simulink model "run_quadrotor_2020a"  (R2020a)
settings: Solver=ode23  StartTime=0.0  StopTime=60  FixedStep=10/1000  MaxStep=0.01  MinStep=1/1000  RelTol=1e-5  EnableMultiTasking=on
InitFcn:
  | addpath('display/')
  | addpath('parameters/')
  | addpath('quadrotor_model')
  | addpath('tools/')
  | addpath('libs/RealTima_Pacer')
  | aerosonde_parameters
  | simulation_parameters
model workspace (MAT data in the model file):
  D1_podbor1 = 902.0676
  D1_podbor_psi = 334.133298018
  D1_podbor_y = 97.9069
  D_podbor_x = 10
  D_podbor_z = 10
  I1_podbor1 = 320.9285
  I1_podbor_psi = 2.71828630961
  I1_podbor_y = 0.6752
  I_podbor_x = 50
  I_podbor_z = 50
  P1_podbor1 = 7509.4
  P1_podbor_psi = 848.547345881
  P1_podbor_y = 264.9363
  P_podbor_x = 50
  P_podbor_z = 50
  theta_1_P_param = Simulink.Parameter
  theta_1_P_param.Value = 1
  theta_1_P_param.DataType = 'auto'
  theta_1_P_param.Dimensions = [1 1]
  theta_1_P_paramCopy = Simulink.Parameter
  theta_1_P_paramCopy.Value = 1
  theta_1_P_paramCopy.DataType = 'auto'
  theta_1_P_paramCopy.Dimensions = [1 1]
undefined symbols (not defined in the file or in its folder): drawQuadrotor, filter_freq, ln, MAV, plotmavstatevariables, setup_pid
libraries: simulink x11, checkpacklib x5, dspsigattribs x2, realtime_pacer_lib x1
(part 1 of 2)
settings Model: PacingRate=0.160000  ParameterArgumentNames=theta_1_P_param  OrderedModelArguments=off  Creator=beard  LastModifiedBy=Tamer
settings SolverCC: ZeroCrossControl=DisableAll
settings DataIOCC: LimitDataPoints=on  SaveFormat=Array  ReturnWorkspaceOutputsName=SDOSimTest_Log
settings OptimizationCC: ExpressionDepthLimit=2147483647  InitFltsAndDblsToZero=on  LifeSpan=inf  SimCompilerOptimization=on
settings DebuggingCC: ReadBeforeWriteMsg=DisableAll  WriteAfterWriteMsg=DisableAll  WriteAfterReadMsg=DisableAll  MergeDetectMultiDrivingBlocksExec=none  SolverPrmCheckMsg=warning  MultiTaskDSMMsg=none  IntegerOverflowMsg=none  FcnCallInpInsideContextMsg=warning  AllowSymbolicDim=off  StateNameClashWarn=warning  SFUnexpectedBacktrackingDiag=warning  SFNoUnconditionalDefaultTransitionDiag=warning  SFExecutionAtInitializationDiag=none  IntegerSaturationMsg=none  ArithmeticOperatorsInVariantConditions=warning
settings ModelReferenceCC: UpdateModelReferenceTargets=IfOutOfDate  PropagateSignalLabelsOutOfModel=off
settings SFSimCC: SFSimEcho=off  SimCtrlC=off  SimUseLocalCustomCode=off  CustomCodeUndefinedFunction=UseInterfaceOnly
settings RTWCC: RTWUseLocalCustomCode=off
settings CodeAppCC: StateflowObjectComments=on
settings GRTTargetCC: TargetLangStandard=C89/C90 (ANSI)  CombineOutputUpdateFcns=off  GRTInterface=on
settings ConfigComp: CovMetricSettings=dw  CovSaveCumulativeToWorkspaceVar=on  CovSaveSingleToWorkspaceVar=on  CovExternalEMLEnable=off  CovSFcnEnable=off

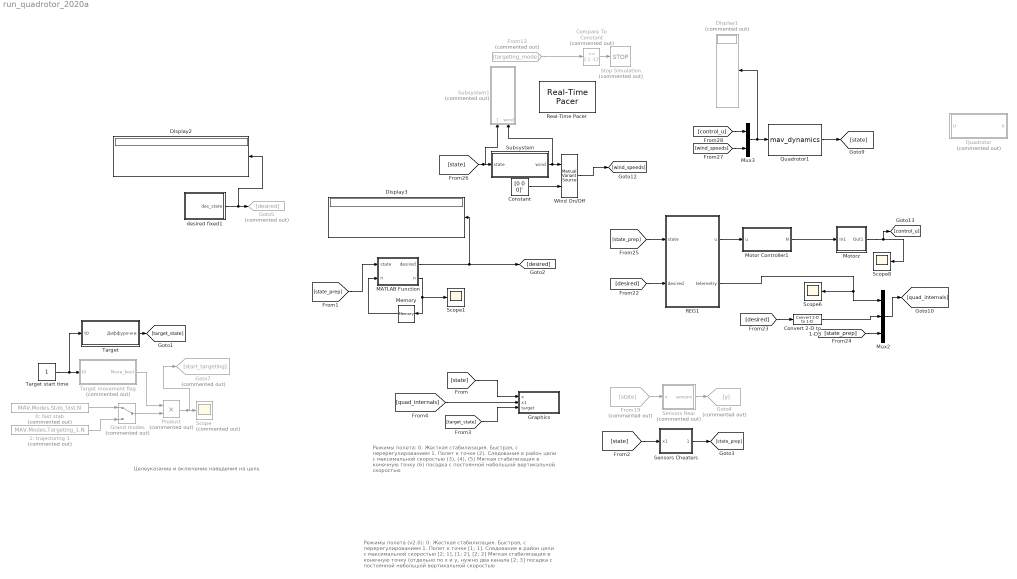
== system run_quadrotor_2020a ==
  note: Целеуказание и включение наведения на цель
  note: Режимы полета:
      | 0. Жесткая стабилизация. Быстрая, с перерегулированием
      | 1. Полет к точке
      |     (2). Следование в район цели с максимальной скоростью
      |     (3), (4), (5) Мягкая стабилизация в конечную точку
      |     (6) посадка с постоянной небольшой вертикальной   скоростью
  note: Режимы полета (v2.0):
      | 0. Жесткая стабилизация. Быстрая, с перерегулированием
      | 1. Полет к точке
      |     [1; 1]. Следование в район цели с максимальной скоростью
      |     [2; 1], [1; 2], [2; 2] Мягкая стабилизация в конечную точку (отдельно по х и у, нужно два канала
      |     [2; 3] посадка с постоянной небольшой вертикальной   скоростью
  0: fast stab : Constant  Commented=on  Value=MAV.Modes.Stab_fast.N
  1: trajectoring 1 : Constant  Commented=on  Value=MAV.Modes.Targeting_1.N
  Compare To Constant : simulink/Logic and Bit Operations/Compare To Constant  Commented=on  relop===  const=[-1 -1]'  OutDataTypeStr=boolean
  Constant : Constant  Value=[0 0 0]'
  Convert 2-D to 1-D3 : dspsigattribs/Convert 2-D to 1-D
      settings: SourceProductBaseCode=DS
  Display1 : Display  Commented=on
  Display2 : Display
  Display3 : Display
  From13 : From  Commented=on  GotoTag=targeting_mode
  From19 : From  Commented=on  GotoTag=state
  Goto4 : Goto  Commented=on  GotoTag=y
  Goto5 : Goto  Commented=on  GotoTag=desired
  Goto7 : Goto  Commented=on  GotoTag=start_targeting
  Grand modes : ManualSwitch  Commented=on
  Graphics : Subsystem
      mask Display: image(imread('../chap2/tv.jpg'))
  MATLAB Function : MATLAB Function  TreatAsAtomicUnit=on
  Memory : Memory
  Motor Controller1 : MATLAB Function  TreatAsAtomicUnit=on
  Motorz : Subsystem
  Mux2 : Mux  Inputs=3
  Mux3 : Mux  Inputs=2
  Product : Product  Commented=on
  Quadrotor : Subsystem  Commented=on
  Quadrotor1 : S-Function  FunctionName=mav_dynamics  Parameters=MAV  SFunctionDeploymentMode=off  EnableBusSupport=off
  REG1 : Subsystem
  Real-Time Pacer : realtime_pacer_lib/Real-Time Pacer  simTimePerRealTime=1
  Scope : Scope  Commented=on
  Scope1 : Scope
  Scope6 : Scope
  Scope8 : Scope
  Sensors Cheaters : Subsystem
  Sensors Real : Subsystem  Commented=on
  Stop Simulation : Stop  Commented=on
  Subsystem : Subsystem
  Subsystem1 : Subsystem  Commented=on
  Target : Subsystem
  Target movement flag : Subsystem  Commented=on
  Target start time : Constant
  Wind On/Off : simulink/Signal Routing/Manual Variant Source  NumChoices=2  LabelModeActiveChoice=V_1
  desired fixed1 : MATLAB Function  TreatAsAtomicUnit=on
  wires:
  Target/1("Диффурочки ") -> [target_state]
  0: fast stab/1 -> Grand modes/1
  1: trajectoring 1/1 -> Grand modes/2
  Grand modes/1 -> Product/2
  Target movement flag/1(Move_bool) -> Product/1
  Product/1 -> Goto7/1, Scope/1
  [state] -> Graphics/1(x)
  [target_state] -> Graphics/3(target)
  Sensors Cheaters/1(sensors) -> [state_prep]
  [quad_internals] -> Graphics/2(x1)
  Compare To Constant/1 -> Stop Simulation/1
  From13/1 -> Compare To Constant/1
  Target start time/1 -> Target/1(t0), Target movement flag/1(t0)
  Sensors Real/1(sensors) -> Goto4/1
  From19/1 -> Sensors Real/1("x ")
  [state] -> Sensors Cheaters/1(x1)
  [state_prep] -> Mux2/3
  [desired] -> Convert 2-D to 1-D3/1
  Mux2/1 -> [quad_internals]
  [desired] -> REG1/2(desired)
  REG1/2(telemetry) -> Mux2/1, Scope6/1
  [state_prep] -> REG1/1(state)
  Convert 2-D to 1-D3/1 -> Mux2/2
  REG1/1(u) -> Motor Controller1/1(u)
  Motor Controller1/1(N) -> Motorz/1(In1)
  Motorz/1(Out1) -> [control_u], Scope8/1
  [state] -> Subsystem1/1(state), Subsystem/1(state)
  Subsystem/1(wind) -> Subsystem1/2(wind), Wind On/Off/1
  [control_u] -> Mux3/1
  [wind_speeds] -> Mux3/2
  Mux3/1 -> Display1/1, Quadrotor1/1
  Quadrotor1/1 -> [state]
  desired fixed1/1(des_state) -> Display2/1, Goto5/1
  Constant/1 -> Wind On/Off/2
  Wind On/Off/1 -> [wind_speeds]
  [state_prep] -> MATLAB Function/1(state)
  MATLAB Function/1(desired) -> Display3/1, [desired]
  MATLAB Function/2(n) -> Scope1/1, Memory/1
  Memory/1 -> MATLAB Function/2("n ")

== system run_quadrotor_2020a/Graphics ==
  note: 2. Дежрать окно с дерьмом в фокусе нахуй мое уважение
  note: 1. Переключиться на другое окно, затем переключить фокус обратно
  note: Attention!!! Для динамического изменения положения камеры (слежение за квадром) необходимо:
  x : Inport
  x1 : Inport  Port=2
  target : Inport  Port=3
  Clock : Clock
  Mux : Mux
  drawQuadrotor : MATLABFcn  MATLABFcn=drawQuadrotor(u)  OutputDimensions=0  SampleTime=0
  plotStateVariables : MATLABFcn  MATLABFcn=plotmavstatevariables(u)  OutputDimensions=0
  wires:
  x/1 -> Mux/1
  Clock/1 -> Mux/4
  x1/1 -> Mux/2
  target/1 -> Mux/3
  Mux/1 -> drawQuadrotor/1, plotStateVariables/1

== system run_quadrotor_2020a/Motorz ==
  In1 : Inport
  Demux : Demux
  Motor{,1..3} (4 alike) : TransferFcn  Denominator=[MAV.Motor.T 1]
  Mux : Mux
  Out1 : Outport
  wires:
  In1/1 -> Demux/1
  Demux/1 -> Motor/1
  Demux/2 -> Motor1/1
  Demux/3 -> Motor2/1
  Demux/4 -> Motor3/1
  Mux/1 -> Out1/1
  Motor/1 -> Mux/1
  Motor1/1 -> Mux/2
  Motor2/1 -> Mux/3
  Motor3/1 -> Mux/4

== system run_quadrotor_2020a/Quadrotor ==
  U : Inport
  Clock : Clock
  Integrator : Integrator  InitialCondition=[MAV.pn0 MAV.pe0 MAV.pd0 MAV.u0 MAV.v0 MAV.w0 MAV.phi0 MAV.theta0 MAV.psi0 MAV.p0 MAV.q0 MAV.r0]'
  MATLAB Function : MATLAB Function  TreatAsAtomicUnit=on
  X : Outport
  wires:
  MATLAB Function/1(y) -> Integrator/1
  Integrator/1 -> X/1, MATLAB Function/2(x)
  U/1 -> MATLAB Function/3(uu)
  Clock/1 -> MATLAB Function/1(t)

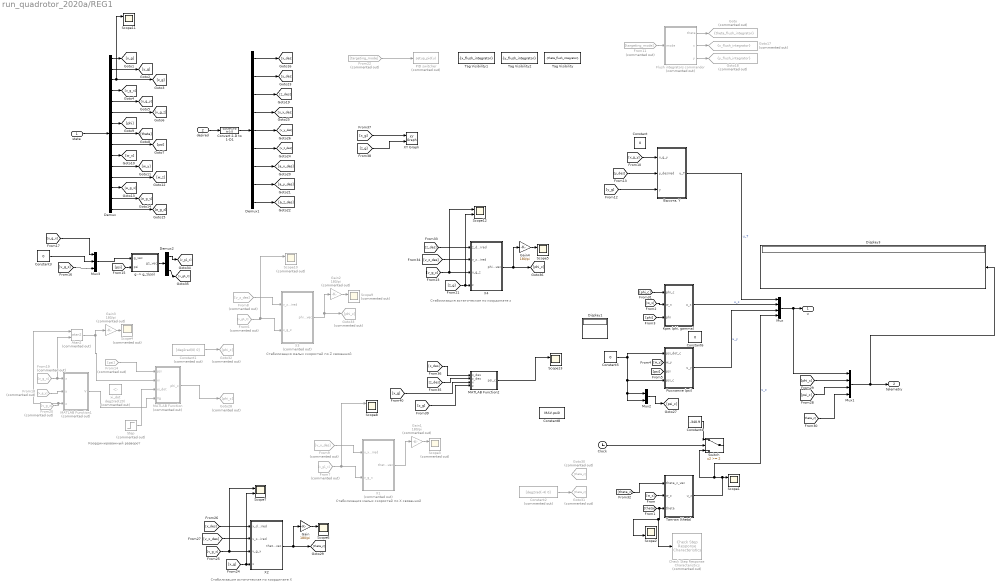
== system run_quadrotor_2020a/REG1 ==
  note: Координированный разворот
  note: Стабилизация астатическая по координате Х
  note: Стабилизация малых скоростей по Х связанной
  note: Стабилизация малых скоростей по Z связанной
  note: Стабилизация астатическая по координате z
  state : Inport
  desired : Inport  Port=2
  Atan2 : Trigonometry  Commented=on  Operator=atan2
  Check Step Response Characteristics : checkpacklib/Check Step Response  Characteristics  Commented=on  InstantiateOnLoad=on  enabled=off  stopWhenAssertionFail=off  export=off  ViewDlgPos=[]  OpenViewOnLoad=off  LaunchViewOnOpen=off  TimeUnits=seconds  EnableStepResponseBound=on  InitialValue=0  FinalValue=-deg2rad(3)  StepTime=0  RiseTime=1.9  PercentRise=80  SettlingTime=2  PercentSettling=1  PercentOvershoot=30  PercentUndershoot=0
      settings: SourceProductBaseCode=CT,ID,MT,SO
  Clock : Clock
  Constant{,3,5..6} (4 alike) : Constant  Value=0
  Constant1 : Constant  Commented=on  Value=[deg2rad(0) 0]
  Constant2 : Constant  Commented=on  Value=[deg2rad(-4) 0]
  Constant4 : Constant  Value=-340.9
  Constant8 : Constant  Value=MAV.psi0
  Convert 2-D to 1-D1 : dspsigattribs/Convert 2-D to 1-D
      settings: SourceProductBaseCode=DS
  Demux : Demux  Outputs=15
  Demux1 : Demux  Outputs=9
  Demux2 : Demux  Outputs=3
  Display1 : Display
  Display3 : Display
  Flush integrators commandor : Subsystem  Commented=on
  From11 : From  Commented=on  GotoTag=targeting_mode  TagVisibility=global
  From14 : From  Commented=on  GotoTag=psi
  From18 : From  Commented=on  GotoTag=v_g_y
  From19 : From  Commented=on  GotoTag=v_g_x
  From20 : From  Commented=on  GotoTag=v_g_z
  From22 : From  Commented=on  GotoTag=targeting_mode  TagVisibility=global
  From6 : From  Commented=on  GotoTag=v_g1_z
  From7 : From  Commented=on  GotoTag=v_g1_x
  From8 : From  Commented=on  GotoTag=v_z_des
  From9 : From  Commented=on  GotoTag=v_x_des
  Gain : Gain  Gain=180/pi
  Gain1 : Gain  Commented=on  Gain=180/pi
  Gain2 : Gain  Commented=on  Gain=180/pi
  Gain3 : Gain  Commented=on  Gain=180/pi
  Gain4 : Gain  Gain=180/pi
  Goto : Goto  Commented=on  GotoTag=theta_flush_integrator  TagVisibility=scoped
  Goto17 : Goto  Commented=on  GotoTag=x_flush_integrator  TagVisibility=scoped
  Goto18 : Goto  Commented=on  GotoTag=y_flush_integrator  TagVisibility=scoped
  Goto28 : Goto  Commented=on  GotoTag=phi_c
  Goto30 : Goto  Commented=on  GotoTag=theta_c
  Goto31 : Goto  Commented=on  GotoTag=theta_c
  Goto32 : Goto  Commented=on  GotoTag=phi_c
  Goto33 : Goto  Commented=on  GotoTag=phi_c
  MATLAB Function : MATLAB Function  Commented=on  TreatAsAtomicUnit=on
  MATLAB Function1 : MATLAB Function  Commented=on  TreatAsAtomicUnit=on
  MATLAB Function2 : MATLAB Function  TreatAsAtomicUnit=on
  Mux : Mux
  Mux1 : Mux
  Mux2 : Mux  Inputs=2
  Mux3 : Mux  Inputs=3
  PID switcher : MATLABFcn  Commented=on  MATLABFcn=setup_pid(u)  OutputDimensions=0  Output1D=off
  Scope{1..2,5..8,11..13} (9 alike) : Scope  NumInputPorts=2
  Scope10 : Scope  Commented=on  NumInputPorts=2
  Scope3 : Scope  Commented=on  NumInputPorts=2
  Scope4 : Scope  Commented=on
  Scope9 : Scope  Commented=on  NumInputPorts=2
  Step : Step  Commented=on  Time=2  After=deg2rad(20)  SampleTime=0
  Switch : Switch  Threshold=2
  Tag Visibility : GotoTagVisibility  GotoTag=theta_flush_integrator
  Tag Visibility1 : GotoTagVisibility  GotoTag=x_flush_integrator
  Tag Visibility2 : GotoTagVisibility  GotoTag=y_flush_integrator
  X1 : Subsystem  Commented=on
  X2 : Subsystem
  X3 : Subsystem  Commented=on
  X4 : Subsystem
  XY Graph : simulink/Sinks/XY Graph  xmin=-40  xmax=40  ymin=-40  ymax=40  st=-1
  "g -> g_1(psi)" : MATLAB Function  TreatAsAtomicUnit=on
  xi_dot : Constant  Commented=on  Value=deg2rad(20)
  "Высота, Y" : Subsystem
      settings: PortSchema="{\"entries\":[{\"content\":{\"sides\":[{\"content\":{\"connectorIds\":[]},\"type\":\"ConnectorPlacement.EquallySpacedRectSide\",\"uuid\":\"a258f665-a86a-4482-bd07-3187ea478656\"},{\"content\":{\"connectorIds\":[],\"side\":\"RIGHT\"},\"type\":\"ConnectorPlacement.EquallySpacedRectSide\",\"uuid\":\"4cc1ffc1-e5d7-4190-ba75-89ce977e4acc\"},{\"content\":{\"connectorIds\":[\"Out1\"],\"side\":\"TOP\"},\"type\":\"ConnectorPlacement.EquallySpacedRectSide\",\"uuid\":\"daf9489c-9fb9-498c-b344-dda7a980194c\"},{\"content\":{\"connectorIds\":[\"In1\",\"In2\",\"In3\"],\"side\":\"BOTTOM\"},\"type\":\"ConnectorPlacement.EquallySpacedRectSide\",\"uuid\":\"f778d476-c858-4cc3-a786-5ff47391ec3b\"}]},\"type\":\"ConnectorPlacement.EquallySpacedConnector\",\"uuid\":\"5a79eedc-deb4-47bd-85cd-0d2cb0ea5802\"}],\"packageUris\":[\"http://schema.mathworks.com/mf0/Connector/19700101\"],\"version\":\"1.0\"}"
  "Крэк (phi, gamma)" : Subsystem
      settings: PortSchema="{\"entries\":[{\"content\":{\"sides\":[{\"content\":{\"connectorIds\":[]},\"type\":\"ConnectorPlacement.EquallySpacedRectSide\",\"uuid\":\"a258f665-a86a-4482-bd07-3187ea478656\"},{\"content\":{\"connectorIds\":[],\"side\":\"RIGHT\"},\"type\":\"ConnectorPlacement.EquallySpacedRectSide\",\"uuid\":\"4cc1ffc1-e5d7-4190-ba75-89ce977e4acc\"},{\"content\":{\"connectorIds\":[\"Out1\"],\"side\":\"TOP\"},\"type\":\"ConnectorPlacement.EquallySpacedRectSide\",\"uuid\":\"daf9489c-9fb9-498c-b344-dda7a980194c\"},{\"content\":{\"connectorIds\":[\"In1\",\"In2\",\"In3\"],\"side\":\"BOTTOM\"},\"type\":\"ConnectorPlacement.EquallySpacedRectSide\",\"uuid\":\"f778d476-c858-4cc3-a786-5ff47391ec3b\"}]},\"type\":\"ConnectorPlacement.EquallySpacedConnector\",\"uuid\":\"5a79eedc-deb4-47bd-85cd-0d2cb0ea5802\"}],\"packageUris\":[\"http://schema.mathworks.com/mf0/Connector/19700101\"],\"version\":\"1.0\"}"
  Рыскание (psi) : Subsystem
      settings: PortSchema="{\"entries\":[{\"content\":{\"sides\":[{\"content\":{\"connectorIds\":[]},\"type\":\"ConnectorPlacement.EquallySpacedRectSide\",\"uuid\":\"a258f665-a86a-4482-bd07-3187ea478656\"},{\"content\":{\"connectorIds\":[],\"side\":\"RIGHT\"},\"type\":\"ConnectorPlacement.EquallySpacedRectSide\",\"uuid\":\"4cc1ffc1-e5d7-4190-ba75-89ce977e4acc\"},{\"content\":{\"connectorIds\":[\"Out1\"],\"side\":\"TOP\"},\"type\":\"ConnectorPlacement.EquallySpacedRectSide\",\"uuid\":\"daf9489c-9fb9-498c-b344-dda7a980194c\"},{\"content\":{\"connectorIds\":[\"In1\",\"In2\",\"In3\",\"In4\"],\"side\":\"BOTTOM\"},\"type\":\"ConnectorPlacement.EquallySpacedRectSide\",\"uuid\":\"f778d476-c858-4cc3-a786-5ff47391ec3b\"}]},\"type\":\"ConnectorPlacement.EquallySpacedConnector\",\"uuid\":\"5a79eedc-deb4-47bd-85cd-0d2cb0ea5802\"}],\"packageUris\":[\"http://schema.mathworks.com/mf0/Connector/19700101\"],\"version\":\"1.0\"}"
  Тангаж (theta) : Subsystem
      settings: PortSchema="{\"entries\":[{\"content\":{\"sides\":[{\"content\":{\"connectorIds\":[]},\"type\":\"ConnectorPlacement.EquallySpacedRectSide\",\"uuid\":\"a258f665-a86a-4482-bd07-3187ea478656\"},{\"content\":{\"connectorIds\":[],\"side\":\"RIGHT\"},\"type\":\"ConnectorPlacement.EquallySpacedRectSide\",\"uuid\":\"4cc1ffc1-e5d7-4190-ba75-89ce977e4acc\"},{\"content\":{\"connectorIds\":[\"Out1\"],\"side\":\"TOP\"},\"type\":\"ConnectorPlacement.EquallySpacedRectSide\",\"uuid\":\"daf9489c-9fb9-498c-b344-dda7a980194c\"},{\"content\":{\"connectorIds\":[\"In1\",\"In2\",\"In3\"],\"side\":\"BOTTOM\"},\"type\":\"ConnectorPlacement.EquallySpacedRectSide\",\"uuid\":\"f778d476-c858-4cc3-a786-5ff47391ec3b\"}]},\"type\":\"ConnectorPlacement.EquallySpacedConnector\",\"uuid\":\"5a79eedc-deb4-47bd-85cd-0d2cb0ea5802\"}],\"packageUris\":[\"http://schema.mathworks.com/mf0/Connector/19700101\"],\"version\":\"1.0\"}"
  u : Outport
  telemetry : Outport  Port=2
  wires:
  From11/1 -> Flush integrators commandor/1(mode)
  Flush integrators commandor/1(theta) -> Goto/1
  Mux/1 -> Mux1/1, u/1
  state/1 -> Demux/1
  Demux/1 -> [x_g]
  Demux/2 -> [y_g]
  Demux/3 -> [z_g], Scope11/1
  Demux/4 -> [v_g_x]
  Demux/5 -> [v_g_y]
  Demux/6 -> [v_g_z]
  Demux/7 -> [phi]
  Demux/8 -> [theta]
  Demux/9 -> [psi]
  Demux/10 -> [w_x]
  Demux/11 -> [w_y]
  Demux/12 -> [w_z]
  Demux/13 -> [a_g_x]
  Demux/14 -> [a_g_y]
  Demux/15 -> [a_g_z]
  [w_z] -> Тангаж (theta)/2(w_z)
  [theta] -> Check Step Response Characteristics/1, Scope2/2, Тангаж (theta)/3(theta)
  Demux1/5 -> [v_y_des]
  Demux1/2 -> [y_des]
  Demux1/4 -> [v_x_des]
  Demux1/1 -> [x_des]
  Flush integrators commandor/2(x) -> Goto17/1
  Flush integrators commandor/3(y) -> Goto18/1
  From22/1 -> PID switcher/1
  Mux1/1 -> Display3/1, telemetry/1
  desired/1 -> Convert 2-D to 1-D1/1
  Convert 2-D to 1-D1/1 -> Demux1/1
  Demux1/9 -> [a_z_des]
  Demux1/7 -> [a_x_des]
  Demux1/8 -> [a_y_des]
  [w_x] -> "Крэк (phi, gamma)"/2(w_x)
  [phi] -> "Крэк (phi, gamma)"/3(phi)
  [w_y] -> Рыскание (psi)/2(w_y)
  [psi] -> Рыскание (psi)/3(psi)
  Constant5/1 -> Рыскание (psi)/4(psi_c), Mux2/1, Mux2/2, Рыскание (psi)/1(psi_dot_c)
  "Крэк (phi, gamma)"/1(u_x) -> Mux/2  "u_x"
  Тангаж (theta)/1(u_z) -> Scope1/1, Mux/4, Switch/3  "u_z"
  MATLAB Function2/1(psi_c) -> Scope13/1
  "Высота, Y"/1(u_T) -> Mux/1  "u_T"
  Demux1/3 -> [z_des]
  Demux1/6 -> [v_z_des]
  [x_des] -> X2/1(x_desired)
  [v_x_des] -> X2/2(v_x_desired)
  [v_g_x] -> Scope7/1, X2/3(v_g_x)
  X2/1(theta_c_vec) -> [theta_c], Gain/1
  [x_g] -> Scope7/2, X2/4(x)
  Mux2/1 -> [psi_c]
  [phi_c] -> Mux1/2
  [psi_c] -> Mux1/3
  [phi_c] -> "Крэк (phi, gamma)"/1(phi_c)
  Constant1/1 -> Goto32/1
  Constant2/1 -> Goto31/1
  [theta_c] -> Mux1/4
  Gain/1 -> Scope6/1
  From7/1 -> Scope8/1, X1/2(v_g_x)
  Gain1/1 -> Scope3/1
  From9/1 -> X1/1(v_x_desired)
  Gain2/1 -> Scope9/1
  X3/1(phi_c_vec) -> Goto33/1, Gain2/1
  From8/1 -> X3/1(v_z_desired)
  From6/1 -> Scope10/1, X3/2(v_g_z)
  [psi] -> "g -> g_1(psi)"/2(psi)
  "g -> g_1(psi)"/1(g1_vec) -> Demux2/1
  Mux3/1 -> "g -> g_1(psi)"/1(g_vec)
  [v_g_z] -> Mux3/3
  Constant3/1 -> Mux3/2
  [v_g_x] -> Mux3/1
  Demux2/1 -> [v_g1_x]
  Demux2/3 -> [v_g1_z]
  [y_g] -> "Высота, Y"/3(y)
  From14/1 -> MATLAB Function/1(psi)
  From19/1 -> Atan2/2, MATLAB Function1/1(x)
  From18/1 -> MATLAB Function1/2(y)
  From20/1 -> Atan2/1, MATLAB Function1/3(z)
  MATLAB Function1/1(V) -> MATLAB Function/4(Vg)
  Atan2/1 -> MATLAB Function/2(xi), Gain3/1
  Gain3/1 -> Scope4/1
  MATLAB Function/1(phi_c) -> Goto28/1
  Step/1 -> MATLAB Function/3(xi_dot)
  Clock/1 -> Switch/2
  Constant4/1 -> Switch/1
  X1/1(theta_c_vec) -> Gain1/1
  ? -> Goto30/1
  [theta_c] -> Тангаж (theta)/1(theta_c_vec)
  [z_des] -> X4/1(z_desired)
  Gain4/1 -> Scope5/1
  [v_z_des] -> X4/2(v_z_desired)
  X4/1(phi_c_vec) -> [phi_c], Gain4/1
  [v_g_z] -> Scope12/1, X4/3(v_g_z)
  [z_g] -> Scope12/2, X4/4(z)
  [y_des] -> "Высота, Y"/2(y_desired)
  [v_g_y] -> "Высота, Y"/1(v_g_y)
  [z_des] -> MATLAB Function2/2(z_des)
  [x_des] -> MATLAB Function2/1(x_des)
  [x_g] -> XY Graph/1
  [z_g] -> XY Graph/2
  [z_g] -> MATLAB Function2/4(z)
  [x_g] -> MATLAB Function2/3(x)
  Рыскание (psi)/1(u_y) -> Mux/3  "u_y"

== system run_quadrotor_2020a/Sensors Cheaters ==
  x1 : Inport
  Constant : Constant  Commented=on  Value=0
  Demux : Demux  Commented=on  Outputs=12
  Demux1 : Demux  Outputs=12
  Derivative{,1..3} (4 alike) : Derivative  Commented=on
  Mux : Mux  Commented=on  Inputs=3
  Mux1 : Mux  Commented=on  Inputs=15
  Mux{2,4..6} (4 alike) : Mux  Inputs=3
  Mux3 : Mux  Inputs=5
  Transfer Fcn2 : TransferFcn  Commented=on  Denominator=[1/filter_freq 1]
  Vg : Derivative
  Vg1 : Derivative
  sensors : Outport
  wires:
  Demux/3 -> Mux1/3
  Constant/1 -> Mux1/6, Mux1/15
  Demux/12 -> Mux1/11  "w_z"
  Demux/10 -> Mux1/10  "w_x"
  Demux/9 -> Mux1/9
  Demux/8 -> Mux1/8
  Demux/7 -> Mux1/7
  Demux/11 -> Mux1/12  "w_y"
  Demux/1 -> Mux1/1, Derivative/1
  Demux/2 -> Mux1/2, Derivative3/1
  Derivative/1 -> Derivative1/1, Mux1/4
  Derivative3/1 -> Derivative2/1, Mux1/5
  Derivative1/1 -> Mux1/13
  Derivative2/1 -> Mux1/14
  Demux1/12 -> Mux5/3  "w_z"
  Mux5/1 -> Mux3/4  "w"
  Mux4/1 -> Mux3/3  "Euler"
  Demux1/10 -> Mux5/1  "w_x"
  Demux1/8 -> Mux4/2  "theta"
  Demux1/7 -> Mux4/1  "phi"
  Demux1/6 -> Mux2/3  "Vz"
  Demux1/9 -> Mux4/3  "psi"
  Demux1/5 -> Mux2/2  "Vy"
  Demux1/4 -> Mux2/1  "Vx"
  Demux1/1 -> Mux6/1  "Xg"
  Demux1/2 -> Mux6/2  "Yg"
  Mux6/1 -> Vg/1, Mux3/1  "Rg"
  Vg/1 -> Mux3/2, Vg1/1
  Vg1/1 -> Mux3/5
  Demux1/3 -> Mux6/3
  Mux3/1 -> sensors/1
  x1/1 -> Demux1/1
  Demux1/11 -> Mux5/2  "w_y"

== system run_quadrotor_2020a/Sensors Real ==
  "x " : Inport
  Demux : Demux  Outputs=12
  MATLAB Function : MATLAB Function  TreatAsAtomicUnit=on
  Mux : Mux  Inputs=3
  Mux1 : Mux  Inputs=2
  Mux2 : Mux  Inputs=3
  Mux3 : Mux  Inputs=3
  v_b_dot : Derivative
  sensors : Outport
  wires:
  "x "/1 -> Demux/1
  Mux1/1 -> sensors/1
  Demux/4 -> Mux/1  "vx"
  Demux/5 -> Mux/2  "vy"
  Demux/6 -> Mux/3  "vz"
  Mux/1 -> MATLAB Function/1(v), v_b_dot/1
  v_b_dot/1 -> MATLAB Function/2(d_v)
  Demux/7 -> Mux2/1  "phi"
  Demux/8 -> Mux2/2  "theta"
  Demux/9 -> Mux2/3  "psi"
  Mux2/1 -> MATLAB Function/3(ang)
  Demux/10 -> Mux3/1  "w_x"
  Demux/11 -> Mux3/2  "w_y"
  Demux/12 -> Mux3/3  "w_z"
  Mux3/1 -> MATLAB Function/4(w), Mux1/2  "gyro"
  MATLAB Function/1(a_prop) -> Mux1/1  "accel"

== system run_quadrotor_2020a/Subsystem ==
  note: Н, м
  state : Inport
  "    Постоянная составляющая скорости ветра < 300 м" : Fcn  Expr=u(1)*((ln(u(2)/0.15)/(ln(u(3)/0.15))))
  Display3 : Display
  Euler : Selector  InputPortWidth=12  IndexOptions=Index vector (dialog)  Indices=[7, 8, 9]  OutputSizes=1
  H : Selector  InputPortWidth=12  IndexOptions=Index vector (dialog)  Indices=[3]  OutputSizes=1
  MinMax : MinMax  Function=max  Inputs=2
  Mux : Mux  Inputs=3
  Scope : Scope
  Subsystem3 : Subsystem
  Vb : Selector  InputPortWidth=12  IndexOptions=Index vector (dialog)  Indices=[4 5 6]  OutputSizes=1
  Высота измерения среднегодовой скорости : Constant  Value=MAV.Env.Wind_speed_h
  Высота измерения среднегодовой скорости1 : Constant  Value=0.5
  "скорость ветра на Н=6 м " : Constant  Value=MAV.Env.Wind_speed_statistics
  wind : Outport
  wires:
  Высота измерения среднегодовой скорости/1 -> Mux/3
  Mux/1 -> "    Постоянная составляющая скорости ветра < 300 м"/1
  "    Постоянная составляющая скорости ветра < 300 м"/1 -> Subsystem3/3(Wind)
  "скорость ветра на Н=6 м "/1 -> Mux/1, Subsystem3/4(V6)
  Vb/1 -> Subsystem3/2(Vb)
  Euler/1 -> Subsystem3/1(euler)
  H/1 -> MinMax/1
  state/1 -> H/1, Vb/1, Euler/1
  Subsystem3/1(wind) -> Scope/1, wind/1
  MinMax/1 -> Display3/1, Subsystem3/5(H), Mux/2
  Высота измерения среднегодовой скорости1/1 -> MinMax/2

== system run_quadrotor_2020a/Subsystem1 ==
  state : Inport
  wind : Inport  Port=2
  "In what the force, bro?" : MATLAB Function  TreatAsAtomicUnit=on
  Old Force : MATLAB Function  TreatAsAtomicUnit=on
  Scope : Scope
  Scope1 : Scope
  Vb : Selector  InputPortWidth=12  IndexOptions=Index vector (dialog)  Indices=[4:6]  OutputSizes=1
  wires:
  state/1 -> Vb/1
  Vb/1 -> Old Force/1(v), "In what the force, bro?"/1(Vb)
  wind/1 -> Old Force/2(w), "In what the force, bro?"/2(Wb)
  "In what the force, bro?"/1(Fb) -> Scope/1
  Old Force/1(F) -> Scope1/1

== system run_quadrotor_2020a/Target ==
  t0 : Inport
  Clock : Clock
  Mux : Mux  Inputs=3
  Mux1 : Mux  Inputs=3
  Mux2 : Mux  Inputs=3
  Scope : Scope
  Target equations : MATLAB Function  TreatAsAtomicUnit=on
  a : Constant  Value=[0 0 0]'
  vx : Constant
  vy : Constant  Value=0
  vz : Constant  Value=0
  x0 : Constant  Value=90
  y0 : Constant  Value=0
  z0 : Constant  Value=0
  "Диффурочки " : Outport
  wires:
  Clock/1 -> Target equations/1(t)
  vx/1 -> Mux1/1
  vy/1 -> Mux1/2
  vz/1 -> Mux1/3
  z0/1 -> Mux/3
  y0/1 -> Mux/2
  x0/1 -> Mux/1
  Mux/1 -> Target equations/3(r0)
  Mux1/1 -> Target equations/4(v0)
  a/1 -> Target equations/5(a0)
  Mux2/1 -> "Диффурочки "/1
  Target equations/2(dr) -> Mux2/2
  Target equations/1(r) -> Scope/1, Mux2/1
  Target equations/3(ddr) -> Mux2/3
  t0/1 -> Target equations/2(t0)

== system run_quadrotor_2020a/Target movement flag ==
  t0 : Inport
  Clock1 : Clock
  Constant2 : Constant  Value=0
  Constant4 : Constant
  Sum : Sum  Inputs=|+-
  Switch : Switch  Criteria=u2 > Threshold
  Move_bool : Outport
  wires:
  Clock1/1 -> Sum/1
  Constant4/1 -> Switch/1
  Sum/1 -> Switch/2
  t0/1 -> Sum/2
  Switch/1 -> Move_bool/1
  Constant2/1 -> Switch/3

== system run_quadrotor_2020a/REG1/Flush integrators commandor ==
  mode : Inport
  Demux : Demux  Outputs=3
  MATLAB Function : MATLAB Function  TreatAsAtomicUnit=on
  Memory : Memory  InitialCondition=[0 0 0]'
  Memory1 : Memory  InitialCondition=[0 0]'
  theta : Outport
  x : Outport  Port=2
  y : Outport  Port=3
  wires:
  mode/1 -> MATLAB Function/1("mode_vec ")
  MATLAB Function/1(command) -> Memory/1, Demux/1
  Memory/1 -> MATLAB Function/3(prev_command)
  Demux/1 -> theta/1
  Demux/2 -> x/1
  Demux/3 -> y/1
  MATLAB Function/2(mode_vec) -> Memory1/1
  Memory1/1 -> MATLAB Function/2(prev_mode_vec)

== system run_quadrotor_2020a/REG1/X1 ==
  note: TODO: обнулять x при смене режима
  note: Стабилизация малой скорости по х
  v_x_desired : Inport
  v_g_x : Inport  Port=2
  "+-1.5 " : Saturate
  +-10 : Saturate  Commented=through  UpperLimit=10  LowerLimit=-10
  -50 ... 50 : Saturate  UpperLimit=deg2rad(50)  LowerLimit=deg2rad(-50)
  Constant : Constant  Value=0
  Gain1 : Gain  Gain=-1
  I : Gain  Gain=6.3529
  Integrator : Integrator  ExternalReset=either
  Mux : Mux  Inputs=2
  P : Gain  Gain=1.1266
  Scope : Scope
  Scope1 : Scope
  Sum : Sum  Inputs=|+-
  Sum1 : Sum  Inputs=++|
  X1 : Subsystem
  theta_c_vec : Outport
  wires:
  P/1 -> Sum1/2
  v_x_desired/1 -> [x_c], Sum/1
  Sum/1 -> Scope/1, +-10/1
  +-10/1 -> P/1, Integrator/1
  -50 ... 50/1 -> Mux/1  "theta_c"
  Mux/1 -> theta_c_vec/1
  I/1 -> Sum1/1, Scope1/1
  Constant/1 -> Mux/2
  Sum1/1 -> Gain1/1  "a_x"
  Gain1/1 -> -50 ... 50/1
  "+-1.5 "/1 -> I/1
  Integrator/1 -> "+-1.5 "/1
  v_g_x/1 -> Sum/2

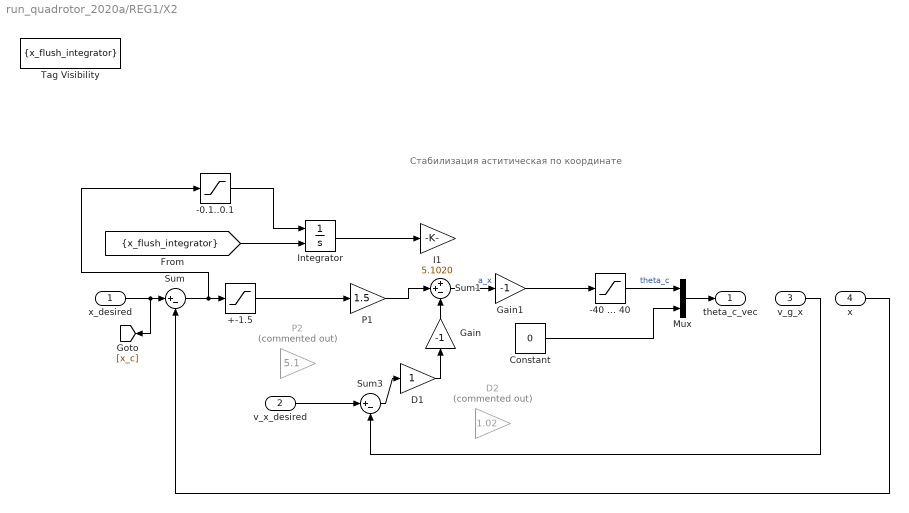
== system run_quadrotor_2020a/REG1/X2 ==
  note: Стабилизация аститическая по координате
  x_desired : Inport
  v_x_desired : Inport  Port=2
  v_g_x : Inport  Port=3
  x : Inport  Port=4
  +-1.5 : Saturate  UpperLimit=1.5  LowerLimit=-1.5
  -0.1..0.1 : Saturate  UpperLimit=0.1  LowerLimit=-0.1
  -40 ... 40 : Saturate  UpperLimit=deg2rad(50)  LowerLimit=deg2rad(-50)
  Constant : Constant  Value=0
  D1 : Gain
  D2 : Gain  Commented=on  Gain=1.02
  Gain : Gain  Gain=-1
  Gain1 : Gain  Gain=-1
  I1 : Gain  Gain=5.1020
  Integrator : Integrator  ExternalReset=either
  Mux : Mux  Inputs=2
  P1 : Gain  Gain=1.5
  P2 : Gain  Commented=on  Gain=5.1
  Sum : Sum  Inputs=|+-
  Sum1 : Sum  Inputs=++-
  Sum3 : Sum  Inputs=|+-
  Tag Visibility : GotoTagVisibility  GotoTag=x_flush_integrator
  theta_c_vec : Outport
  wires:
  P1/1 -> Sum1/2
  x_desired/1 -> [x_c], Sum/1
  D1/1 -> Gain/1
  Sum3/1 -> D1/1
  v_x_desired/1 -> Sum3/1
  v_g_x/1 -> Sum3/2
  [x_flush_integrator] -> Integrator/2
  Gain/1 -> Sum1/3
  Sum/1 -> -0.1..0.1/1, +-1.5/1
  x/1 -> Sum/2
  +-1.5/1 -> P1/1
  -40 ... 40/1 -> Mux/1  "theta_c"
  Mux/1 -> theta_c_vec/1
  Constant/1 -> Mux/2
  Sum1/1 -> Gain1/1  "a_x"
  Gain1/1 -> -40 ... 40/1
  Integrator/1 -> I1/1
  -0.1..0.1/1 -> Integrator/1

== system run_quadrotor_2020a/REG1/X3 ==
  note: TODO: обнулять x при смене режима
  note: Стабилизация малой скорости по z
  v_z_desired : Inport
  v_g_z : Inport  Port=2
  "+-1.5 " : Saturate
  +-10 : Saturate  Commented=through  UpperLimit=10  LowerLimit=-10
  -50 ... 50 : Saturate  UpperLimit=deg2rad(50)  LowerLimit=deg2rad(-50)
  Constant : Constant  Value=0
  I : Gain  Gain=2.8244
  Integrator : Integrator  ExternalReset=either
  Mux : Mux  Inputs=2
  P : Gain  Gain=0.7512
  Scope : Scope
  Scope1 : Scope
  Sum : Sum  Inputs=|+-
  Sum1 : Sum  Inputs=++|
  X1 : Subsystem
  phi_c_vec : Outport
  wires:
  P/1 -> Sum1/2
  v_z_desired/1 -> [x_c], Sum/1
  Sum/1 -> Scope/1, +-10/1
  +-10/1 -> P/1, Integrator/1
  -50 ... 50/1 -> Mux/1  "phi_c"
  Mux/1 -> phi_c_vec/1
  I/1 -> Sum1/1, Scope1/1
  Constant/1 -> Mux/2
  Sum1/1 -> -50 ... 50/1  "a_z"
  "+-1.5 "/1 -> I/1
  Integrator/1 -> "+-1.5 "/1
  v_g_z/1 -> Sum/2

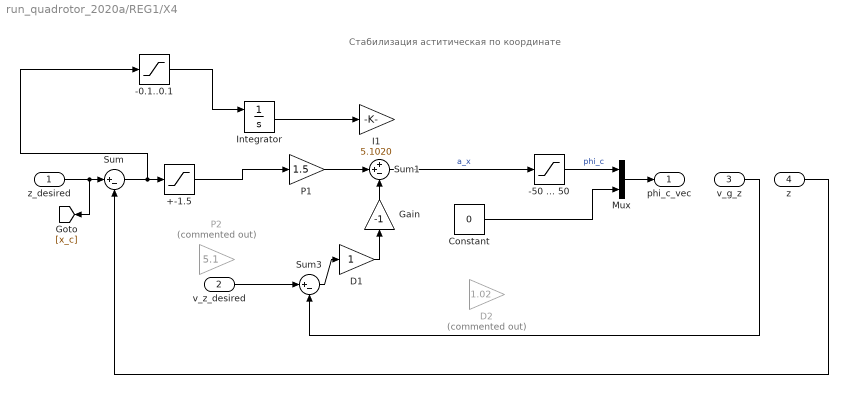
== system run_quadrotor_2020a/REG1/X4 ==
  note: Стабилизация аститическая по координате
  z_desired : Inport
  v_z_desired : Inport  Port=2
  v_g_z : Inport  Port=3
  z : Inport  Port=4
  +-1.5 : Saturate  UpperLimit=1.5  LowerLimit=-1.5
  -0.1..0.1 : Saturate  UpperLimit=0.1  LowerLimit=-0.1
  -50 ... 50 : Saturate  UpperLimit=deg2rad(50)  LowerLimit=deg2rad(-50)
  Constant : Constant  Value=0
  D1 : Gain
  D2 : Gain  Commented=on  Gain=1.02
  Gain : Gain  Gain=-1
  I1 : Gain  Gain=5.1020
  Integrator : Integrator  ExternalReset=either
  Mux : Mux  Inputs=2
  P1 : Gain  Gain=1.5
  P2 : Gain  Commented=on  Gain=5.1
  Sum : Sum  Inputs=|+-
  Sum1 : Sum  Inputs=++-
  Sum3 : Sum  Inputs=|+-
  phi_c_vec : Outport
  wires:
  P1/1 -> Sum1/2
  z_desired/1 -> [x_c], Sum/1
  D1/1 -> Gain/1
  Sum3/1 -> D1/1
  v_z_desired/1 -> Sum3/1
  v_g_z/1 -> Sum3/2
  Gain/1 -> Sum1/3
  Sum/1 -> -0.1..0.1/1, +-1.5/1
  z/1 -> Sum/2
  +-1.5/1 -> P1/1
  -50 ... 50/1 -> Mux/1  "phi_c"
  Mux/1 -> phi_c_vec/1
  Constant/1 -> Mux/2
  Sum1/1 -> -50 ... 50/1  "a_x"
  Integrator/1 -> I1/1
  -0.1..0.1/1 -> Integrator/1

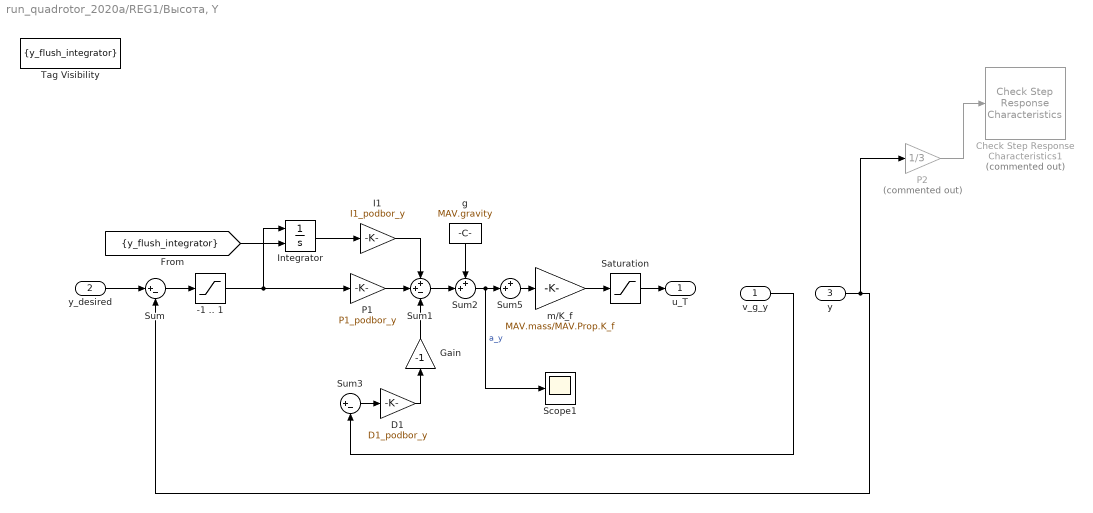
== system run_quadrotor_2020a/REG1/Высота, Y ==
  v_g_y : Inport
  y_desired : Inport  Port=2
  y : Inport  Port=3
  -1 .. 1 : Saturate  UpperLimit=1  LowerLimit=-1
  Check Step Response Characteristics1 : checkpacklib/Check Step Response  Characteristics  Commented=on  InstantiateOnLoad=on  enabled=off  stopWhenAssertionFail=off  export=off  ViewDlgPos=[299 89 1306 720]  OpenViewOnLoad=off  LaunchViewOnOpen=off  TimeUnits=seconds  EnableStepResponseBound=on  InitialValue=0  FinalValue=1  StepTime=1  RiseTime=0.7  PercentRise=80  SettlingTime=1  PercentSettling=1  PercentOvershoot=10  PercentUndershoot=1
      settings: SourceProductBaseCode=CT,ID,MT,SO
  D1 : Gain  Gain=D1_podbor_y
  Gain : Gain  Gain=-1
  I1 : Gain  Gain=I1_podbor_y
  Integrator : Integrator  ExternalReset=either
  P1 : Gain  Gain=P1_podbor_y
  P2 : Gain  Commented=on  Gain=1/3
  Saturation : Saturate  UpperLimit=4*(MAV.Motor.Nmax*0.5)^2  LowerLimit=0
  Scope1 : Scope
  Sum : Sum  Inputs=|+-
  Sum1 : Sum  Inputs=++-
  Sum2 : Sum  Inputs=++|
  Sum3 : Sum  Inputs=|+-
  Sum5 : Sum  Inputs=++|
  Tag Visibility : GotoTagVisibility  GotoTag=y_flush_integrator
  g : Constant  Value=MAV.gravity
  m/K_f : Gain  Gain=MAV.mass/MAV.Prop.K_f
  u_T : Outport
  wires:
  Integrator/1 -> I1/1
  I1/1 -> Sum1/1
  P1/1 -> Sum1/2
  v_g_y/1 -> Sum3/2
  Sum1/1 -> Sum2/2
  g/1 -> Sum2/1
  m/K_f/1 -> Saturation/1
  Saturation/1 -> u_T/1
  Sum3/1 -> D1/1
  D1/1 -> Gain/1
  [y_flush_integrator] -> Integrator/2
  Gain/1 -> Sum1/3
  Sum/1 -> -1 .. 1/1
  -1 .. 1/1 -> P1/1, Integrator/1
  y_desired/1 -> Sum/1
  y/1 -> P2/1, Sum/2
  P2/1 -> Check Step Response Characteristics1/1
  Sum2/1 -> Scope1/1, Sum5/2  "a_y"
  Sum5/1 -> m/K_f/1

== system run_quadrotor_2020a/REG1/Крэк (phi, gamma) ==
  phi_c : Inport
  w_x : Inport  Port=2
  phi : Inport  Port=3
  Check Step Response Characteristics1 : checkpacklib/Check Step Response  Characteristics  Commented=on  InstantiateOnLoad=on  enabled=off  stopWhenAssertionFail=off  export=off  ViewDlgPos=[358 -116 1306 720]  OpenViewOnLoad=off  LaunchViewOnOpen=off  TimeUnits=seconds  EnableStepResponseBound=on  InitialValue=0  FinalValue=1  StepTime=1  RiseTime=0.2  PercentRise=80  SettlingTime=0.5  PercentSettling=1  PercentOvershoot=10  PercentUndershoot=1
      settings: SourceProductBaseCode=CT,ID,MT,SO
  D1 : Gain  Gain=8.6001e+07
  Demux : Demux  Outputs=2
  Divide : Product  Commented=on  Inputs=*/
  Gain : Gain  Gain=-1
  P1 : Gain  Gain=2.5149e+09
  PID Controller : simulink/Continuous/PID Controller  Commented=on  Controller=PID  Form=Parallel  TimeDomain=Continuous-time  UseExternalTs=off  SampleTime=-1  IntegratorMethod=Forward Euler  FilterMethod=Forward Euler  ControllerParametersSource=internal  P=1  I=1  D=0  UseFilter=on  N=100  TunerSelectOption=Transfer Function Based (PID Tuner App)  InitialConditionSource=internal  InitialConditionForIntegrator=0  InitialConditionForFilter=0  DifferentiatorICPrevScaledInput=0  ExternalReset=none  TrackingMode=off  Kt=1  LimitOutput=off  UpperSaturationLimit=inf  LowerSaturationLimit=-inf  LinearizeAsGain=on  AntiWindupMode=none  Kb=1  POutMin=[]  POutMax=[]  IOutMin=[]  IOutMax=[]  DOutMin=[]  DOutMax=[]  NOutMin=[]  NOutMax=[]  SumOutMin=[]  SumOutMax=[]  SaturationOutMin=[]  SaturationOutMax=[]  PParamMin=[]  PParamMax=[]  IParamMin=[]  IParamMax=[]  DParamMin=[]  DParamMax=[]  NParamMin=[]  NParamMax=[]  KbParamMin=[]  KbParamMax=[]  KtParamMin=[]  KtParamMax=[]  KbOutMin=[]  KbOutMax=[]  KtOutMin=[]  KtOutMax=[]  IntegratorOutMin=[]  IntegratorOutMax=[]  FilterOutMin=[]  FilterOutMax=[]  SumI1OutMin=[]  SumI1OutMax=[]  SumI2OutMin=[]  SumI2OutMax=[]  SumI3OutMin=[]  SumI3OutMax=[]  SumI4OutMin=[]  SumI4OutMax=[]  SumDOutMin=[]  SumDOutMax=[]  DifferentiatorOutMin=[]  DifferentiatorOutMax=[]  FilterDiffOutCoefMin=[]  FilterDiffOutCoefMax=[]  ReciprocalOutMin=[]  ReciprocalOutMax=[]  SumDenOutMin=[]  SumDenOutMax=[]  SumNumOutMin=[]  SumNumOutMax=[]  DivideOutMin=[]  DivideOutMax=[]  UdiffTsProdOutMin=[]  UdiffTsProdOutMax=[]  NTsProdOutMin=[]  NTsProdOutMax=[]  UintegralTsProdOutMin=[]  UintegralTsProdOutMax=[]  UngainTsProdOutMin=[]  UngainTsProdOutMax=[]  IntegratorContinuousStateAttributes=''  IntegratorStateMustResolveToSignalObject=off  IntegratorRTWStateStorageClass=Auto  FilterContinuousStateAttributes=''  FilterStateMustResolveToSignalObject=off  FilterRTWStateStorageClass=Auto  ParallelPVariant=InternalParameters  IdealPVariant=Disabled  IVariant=InternalParameters  DVariant=InternalParameters  IntegratorVariant=Continuous  SatVariant=Disabled  AWVariant=Passthrough  PCopyVariant=Disabled  TRVariant=Disabled  FdbkBlocksVariant=Forward  IdealPFdbkVariant=Disabled  SatFdbkVariant=Disabled  DerivativeFilterVariant=ContFilter  NVariant=InternalParameters  NCopyVariant=Disabled  FilterICVariant=InternalICsFilter  IntegratorICVariant=InternalICs  ExternalResetVariant=Disabled  TRSumVariant=Passthrough  SumFdbkVariant=Disabled  SumVariant=Sum_PID  TsampFilterVariant=InternalTs  TsampNgainVariant=Passthrough  TsampIntegralVariant=Passthrough
  Saturation : Saturate  UpperLimit=MAV.Control.u_xz_max  LowerLimit=-MAV.Control.u_xz_max
  Saturation1 : Saturate  UpperLimit=deg2rad(50)  LowerLimit=-deg2rad(50)
  Scope2 : Scope  NumInputPorts=2
  Sum : Sum  Inputs=|+-
  Sum1 : Sum  Inputs=++-
  Sum2 : Sum  Inputs=|+-
  Tag Visibility : GotoTagVisibility  GotoTag=phi_flush_integrator
  u_x : Outport
  wires:
  P1/1 -> Sum1/2
  Sum1/1 -> Saturation/1, Scope2/2  "theta_ddot"
  phi/1 -> Sum/2, Divide/1
  Saturation/1 -> Scope2/1, u_x/1
  Sum2/1 -> D1/1
  D1/1 -> Gain/1
  w_x/1 -> Sum2/2
  Gain/1 -> Sum1/3
  Divide/1 -> Check Step Response Characteristics1/1
  Sum/1 -> P1/1
  Demux/2 -> Sum2/1
  phi_c/1 -> Demux/1
  Demux/1 -> Saturation1/1
  Saturation1/1 -> Sum/1

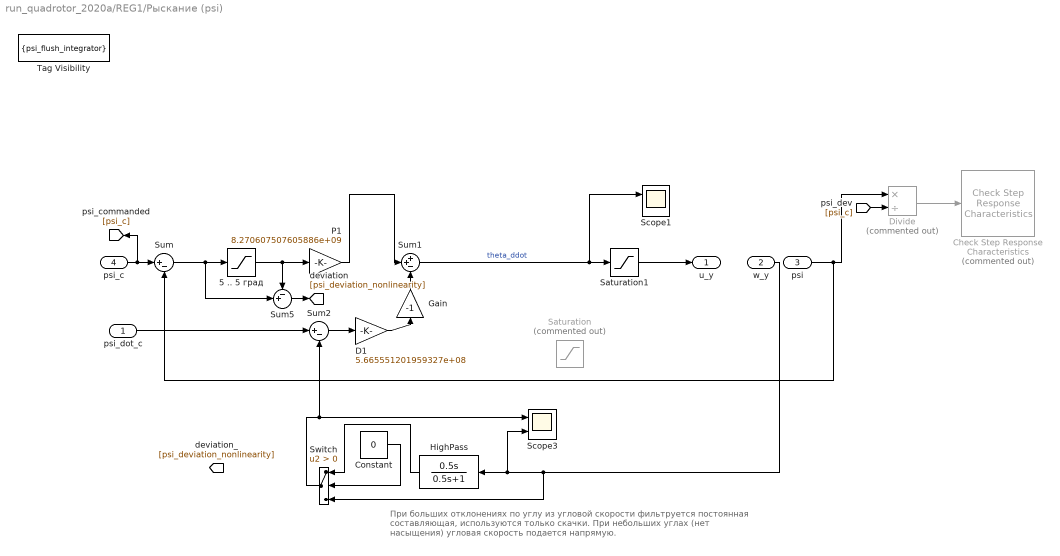
== system run_quadrotor_2020a/REG1/Рыскание (psi) ==
  note: При больших отклонениях по углу из угловой скорости фильтруется
      | постоянная составляющая, используются только скачки.
      | При небольших углах (нет насыщения) угловая скорость подается напрямую.
  psi_dot_c : Inport
  w_y : Inport  Port=2
  psi : Inport  Port=3
  psi_c : Inport  Port=4
  5 .. 5 град : Saturate  UpperLimit=deg2rad(5)  LowerLimit=-deg2rad(5)
  Check Step Response Characteristics : checkpacklib/Check Step Response  Characteristics  Commented=on  InstantiateOnLoad=on  enabled=on  stopWhenAssertionFail=off  export=off  ViewDlgPos=[100 11 1618 919]  OpenViewOnLoad=off  LaunchViewOnOpen=off  TimeUnits=seconds  EnableStepResponseBound=on  InitialValue=0  FinalValue=1  StepTime=1  RiseTime=0.8  PercentRise=80  SettlingTime=1  PercentSettling=1  PercentOvershoot=4  PercentUndershoot=1
      settings: SourceProductBaseCode=CT,ID,MT,SO
  Constant : Constant  Value=0
  D1 : Gain  Gain=5.665551201959327e+08
  Divide : Product  Commented=on  Inputs=*/
  Gain : Gain  Gain=-1
  HighPass : TransferFcn  Numerator=[0.5 0]  Denominator=[0.5 1]
  P1 : Gain  Gain=8.270607507605886e+09
  Saturation : Saturate  Commented=on  UpperLimit=449800000  LowerLimit=-449800000
  Saturation1 : Saturate  UpperLimit=449800000  LowerLimit=-449800000
  Scope1 : Scope  NumInputPorts=2
  Scope3 : Scope  NumInputPorts=2
  Sum : Sum  Inputs=|+-
  Sum1 : Sum  Inputs=++-
  Sum2 : Sum  Inputs=|+-
  Sum5 : Sum  Inputs=-+|
  Switch : Switch  Criteria=u2 > Threshold
  Tag Visibility : GotoTagVisibility  GotoTag=psi_flush_integrator
  u_y : Outport
  wires:
  Sum1/1 -> Saturation1/1, Scope1/1  "theta_ddot"
  psi/1 -> Divide/1, Sum/2
  Saturation1/1 -> u_y/1
  Sum2/1 -> D1/1
  D1/1 -> Gain/1
  Divide/1 -> Check Step Response Characteristics/1
  psi_c/1 -> [psi_c], Sum/1
  psi_dot_c/1 -> Sum2/1
  Sum/1 -> Sum5/2, 5 .. 5 град/1
  5 .. 5 град/1 -> P1/1, Sum5/1
  w_y/1 -> Switch/3, Scope3/2, HighPass/1
  Switch/1 -> Scope3/1, Sum2/2
  Sum5/1 -> [psi_deviation_nonlinearity]
  [psi_c] -> Divide/2
  Gain/1 -> Sum1/3
  P1/1 -> Sum1/2
  Constant/1 -> Switch/2
  HighPass/1 -> Switch/1

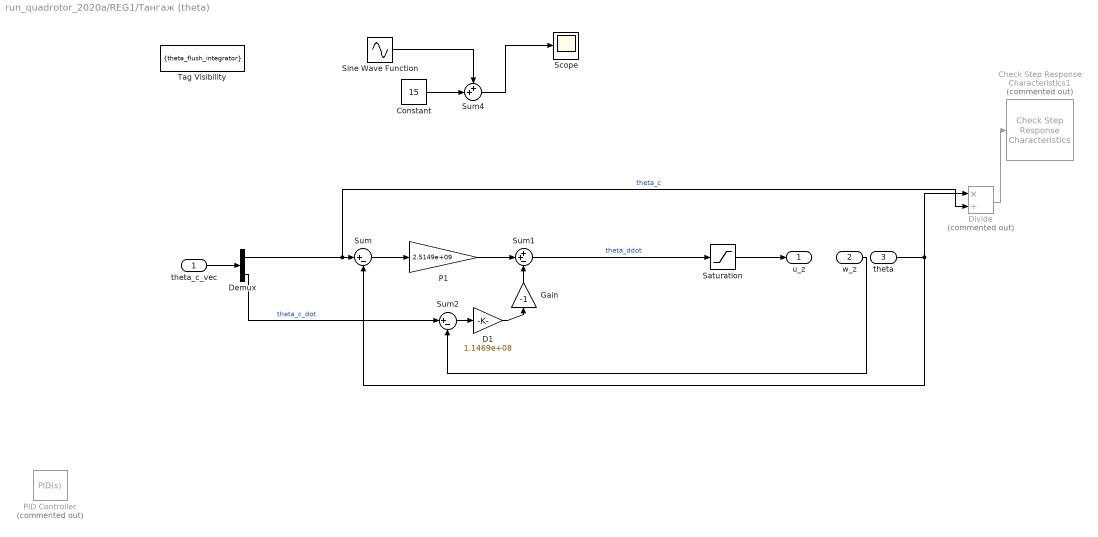
== system run_quadrotor_2020a/REG1/Тангаж (theta) ==
  theta_c_vec : Inport
  w_z : Inport  Port=2
  theta : Inport  Port=3
  Check Step Response Characteristics1 : checkpacklib/Check Step Response  Characteristics  Commented=on  InstantiateOnLoad=on  enabled=off  stopWhenAssertionFail=off  export=off  ViewDlgPos=[435 71 1306 720]  OpenViewOnLoad=off  LaunchViewOnOpen=off  TimeUnits=seconds  EnableStepResponseBound=on  InitialValue=0  FinalValue=1  StepTime=1  RiseTime=0.2  PercentRise=80  SettlingTime=0.5  PercentSettling=1  PercentOvershoot=10  PercentUndershoot=1
      settings: SourceProductBaseCode=CT,ID,MT,SO
  Constant : Constant  Value=15
  D1 : Gain  Gain=1.1469e+08
  Demux : Demux  Outputs=2
  Divide : Product  Commented=on  Inputs=*/
  Gain : Gain  Gain=-1
  P1 : Gain  Gain=2.5149e+09
  PID Controller : simulink/Continuous/PID Controller  Commented=on  Controller=PID  Form=Parallel  TimeDomain=Continuous-time  UseExternalTs=off  SampleTime=-1  IntegratorMethod=Forward Euler  FilterMethod=Forward Euler  ControllerParametersSource=internal  P=1  I=1  D=0  UseFilter=on  N=100  TunerSelectOption=Transfer Function Based (PID Tuner App)  InitialConditionSource=internal  InitialConditionForIntegrator=0  InitialConditionForFilter=0  DifferentiatorICPrevScaledInput=0  ExternalReset=none  TrackingMode=off  Kt=1  LimitOutput=off  UpperSaturationLimit=inf  LowerSaturationLimit=-inf  LinearizeAsGain=on  AntiWindupMode=none  Kb=1  POutMin=[]  POutMax=[]  IOutMin=[]  IOutMax=[]  DOutMin=[]  DOutMax=[]  NOutMin=[]  NOutMax=[]  SumOutMin=[]  SumOutMax=[]  SaturationOutMin=[]  SaturationOutMax=[]  PParamMin=[]  PParamMax=[]  IParamMin=[]  IParamMax=[]  DParamMin=[]  DParamMax=[]  NParamMin=[]  NParamMax=[]  KbParamMin=[]  KbParamMax=[]  KtParamMin=[]  KtParamMax=[]  KbOutMin=[]  KbOutMax=[]  KtOutMin=[]  KtOutMax=[]  IntegratorOutMin=[]  IntegratorOutMax=[]  FilterOutMin=[]  FilterOutMax=[]  SumI1OutMin=[]  SumI1OutMax=[]  SumI2OutMin=[]  SumI2OutMax=[]  SumI3OutMin=[]  SumI3OutMax=[]  SumI4OutMin=[]  SumI4OutMax=[]  SumDOutMin=[]  SumDOutMax=[]  DifferentiatorOutMin=[]  DifferentiatorOutMax=[]  FilterDiffOutCoefMin=[]  FilterDiffOutCoefMax=[]  ReciprocalOutMin=[]  ReciprocalOutMax=[]  SumDenOutMin=[]  SumDenOutMax=[]  SumNumOutMin=[]  SumNumOutMax=[]  DivideOutMin=[]  DivideOutMax=[]  UdiffTsProdOutMin=[]  UdiffTsProdOutMax=[]  NTsProdOutMin=[]  NTsProdOutMax=[]  UintegralTsProdOutMin=[]  UintegralTsProdOutMax=[]  UngainTsProdOutMin=[]  UngainTsProdOutMax=[]  IntegratorContinuousStateAttributes=''  IntegratorStateMustResolveToSignalObject=off  IntegratorRTWStateStorageClass=Auto  FilterContinuousStateAttributes=''  FilterStateMustResolveToSignalObject=off  FilterRTWStateStorageClass=Auto  ParallelPVariant=InternalParameters  IdealPVariant=Disabled  IVariant=InternalParameters  DVariant=InternalParameters  IntegratorVariant=Continuous  SatVariant=Disabled  AWVariant=Passthrough  PCopyVariant=Disabled  TRVariant=Disabled  FdbkBlocksVariant=Forward  IdealPFdbkVariant=Disabled  SatFdbkVariant=Disabled  DerivativeFilterVariant=ContFilter  NVariant=InternalParameters  NCopyVariant=Disabled  FilterICVariant=InternalICsFilter  IntegratorICVariant=InternalICs  ExternalResetVariant=Disabled  TRSumVariant=Passthrough  SumFdbkVariant=Disabled  SumVariant=Sum_PID  TsampFilterVariant=InternalTs  TsampNgainVariant=Passthrough  TsampIntegralVariant=Passthrough
  Saturation : Saturate  UpperLimit=MAV.Control.u_xz_max  LowerLimit=-MAV.Control.u_xz_max
  Scope : Scope
  Sine Wave Function : Sin  Amplitude=15  Frequency=2*pi*1  Phase=2*pi*0.1  SampleTime=0
  Sum : Sum  Inputs=|+-
  Sum1 : Sum  Inputs=++-
  Sum2 : Sum  Inputs=|+-
  Sum4 : Sum  Inputs=++|
  Tag Visibility : GotoTagVisibility  GotoTag=theta_flush_integrator
  u_z : Outport
  wires:
  Sum/1 -> P1/1
  P1/1 -> Sum1/2
  Sum1/1 -> Saturation/1  "theta_ddot"
  theta/1 -> Sum/2, Divide/1
  Saturation/1 -> u_z/1
  Sum2/1 -> D1/1
  D1/1 -> Gain/1
  w_z/1 -> Sum2/2
  Demux/2 -> Sum2/1  "theta_c_dot"
  Divide/1 -> Check Step Response Characteristics1/1
  Sine Wave Function/1 -> Sum4/1
  Constant/1 -> Sum4/2
  Sum4/1 -> Scope/1
  Demux/1 -> Divide/2, Sum/1  "theta_c"
  theta_c_vec/1 -> Demux/1
  Gain/1 -> Sum1/3

== system run_quadrotor_2020a/Subsystem/Subsystem3 ==
  euler : Inport
  Vb : Inport  Port=2
  Wind : Inport  Port=3
  V6 : Inport  Port=4
  H : Inport  Port=5
  Dot Product : DotProduct  InputSameDT=on  OutDataTypeStr=Inherit: Inherit via internal rule
  MATLAB Function1 : MATLAB Function  TreatAsAtomicUnit=on
  Mux : Mux  Inputs=3
  Random Number2 : RandomNumber  SampleTime=0.1
  Sqrt : Sqrt  SaturateOnIntegerOverflow=on
  Sum : Sum  Inputs=|++
  Sum1 : Sum  Inputs=-+|
  Wx1 : Scope
  X1 : Subsystem  TreatAsAtomicUnit=on
  Y2 : Subsystem  TreatAsAtomicUnit=on
  Z1 : Subsystem  TreatAsAtomicUnit=on
  wind : Outport
  wires:
  euler/1 -> MATLAB Function1/1(euler)
  Wind/1 -> MATLAB Function1/2(va)
  MATLAB Function1/1(Wb) -> Sum/1, Sum1/1
  Mux/1 -> Sum/2
  Sum/1 -> wind/1
  Sqrt/1 -> Wx1/1, Y2/2(Va), Z1/3(Va), X1/3(Va)  "Va"
  H/1 -> Y2/1(H), X1/1(H), Z1/1(H)
  V6/1 -> X1/2(V6), Y2/3(V6), Z1/2(V6)
  Z1/1(Out1) -> Mux/3
  X1/1(Out1) -> Mux/1
  Y2/1(Out1) -> Mux/2
  Random Number2/1 -> Y2/4(noise), X1/4(noise), Z1/4(noise)
  Vb/1 -> Sum1/2
  Sum1/1 -> Dot Product/1, Dot Product/2
  Dot Product/1 -> Sqrt/1

== system run_quadrotor_2020a/REG1/X1/X1 ==
  note: TODO: обнулять x при смене режима
  note: Стабилизация малой скорости по х
  v_x_desired : Inport
  x_desired : Inport  Port=2
  v_g_x : Inport  Port=3
  x : Inport  Port=4
  "+-1.5 " : Saturate  UpperLimit=1.5  LowerLimit=-1.5
  +-10 : Saturate  UpperLimit=10  LowerLimit=-10
  -50 ... 50 : Saturate  UpperLimit=deg2rad(50)  LowerLimit=deg2rad(-50)
  Constant : Constant  Value=0
  Gain1 : Gain  Gain=-1
  I : Gain  Gain=5.1020
  Mux : Mux  Inputs=2
  P : Gain  Gain=5.1
  Sum : Sum  Inputs=|+-
  Sum1 : Sum  Inputs=++|
  Sum2 : Sum  Inputs=-+|
  theta_c_vec : Outport
  wires:
  P/1 -> Sum1/2
  v_x_desired/1 -> [x_c], Sum/1
  Sum/1 -> +-10/1
  +-10/1 -> P/1
  -50 ... 50/1 -> Mux/1  "theta_c"
  Mux/1 -> theta_c_vec/1
  I/1 -> Sum1/1
  Constant/1 -> Mux/2
  Sum1/1 -> Gain1/1  "a_x"
  Gain1/1 -> -50 ... 50/1
  "+-1.5 "/1 -> I/1
  Sum2/1 -> "+-1.5 "/1
  x_desired/1 -> Sum2/2
  x/1 -> Sum2/1
  v_g_x/1 -> Sum/2

== system run_quadrotor_2020a/REG1/X3/X1 ==
  note: TODO: обнулять x при смене режима
  note: Стабилизация малой скорости по х
  v_x_desired : Inport
  x_desired : Inport  Port=2
  v_g_x : Inport  Port=3
  x : Inport  Port=4
  "+-1.5 " : Saturate  UpperLimit=1.5  LowerLimit=-1.5
  +-10 : Saturate  UpperLimit=10  LowerLimit=-10
  -50 ... 50 : Saturate  UpperLimit=deg2rad(50)  LowerLimit=deg2rad(-50)
  Constant : Constant  Value=0
  Gain1 : Gain  Gain=-1
  I : Gain  Gain=5.1020
  Mux : Mux  Inputs=2
  P : Gain  Gain=5.1
  Sum : Sum  Inputs=|+-
  Sum1 : Sum  Inputs=++|
  Sum2 : Sum  Inputs=-+|
  theta_c_vec : Outport
  wires:
  P/1 -> Sum1/2
  v_x_desired/1 -> [x_c], Sum/1
  Sum/1 -> +-10/1
  +-10/1 -> P/1
  -50 ... 50/1 -> Mux/1  "theta_c"
  Mux/1 -> theta_c_vec/1
  I/1 -> Sum1/1
  Constant/1 -> Mux/2
  Sum1/1 -> Gain1/1  "a_x"
  Gain1/1 -> -50 ... 50/1
  "+-1.5 "/1 -> I/1
  Sum2/1 -> "+-1.5 "/1
  x_desired/1 -> Sum2/2
  x/1 -> Sum2/1
  v_g_x/1 -> Sum/2

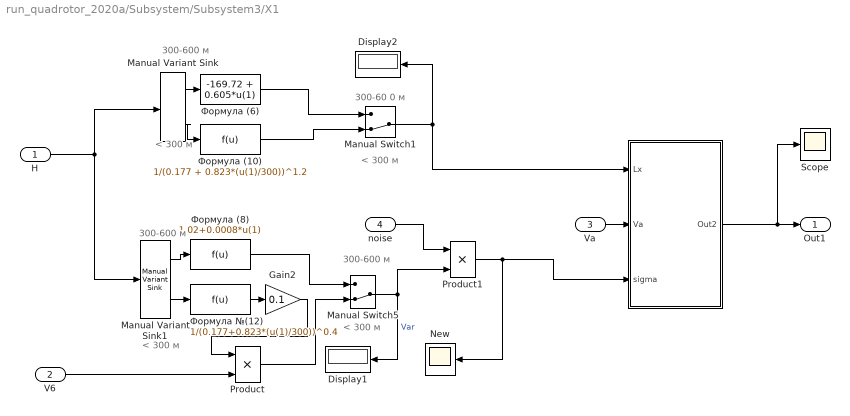
== system run_quadrotor_2020a/Subsystem/Subsystem3/X1 ==
  note: < 300 м
  note: 300-600 м
  note: < 300 м
  note: < 300 м
  note: 300-600 м
  note: < 300 м
  note: 300-60 0 м
  note: 300-600 м
  H : Inport
  V6 : Inport  Port=2
  Va : Inport  Port=3
  noise : Inport  Port=4
  " " : Subsystem
  Display1 : Display
  Display2 : Display
  Gain2 : Gain  Gain=0.1
  Manual Variant Sink : simulink/Signal Routing/Manual Variant Sink  NumChoices=2  LabelModeActiveChoice=V_2
  Manual Variant Sink1 : simulink/Signal Routing/Manual Variant Sink  NumChoices=2  LabelModeActiveChoice=V_2
  Manual Switch1 : ManualSwitch  CurrentSetting=0
  Manual Switch5 : ManualSwitch  CurrentSetting=0
  New : Scope
  Product : Product
  Product1 : Product
  Scope : Scope
  Формула (10) : Fcn  Expr=1/(0.177 + 0.823*(u(1)/300))^1.2
  Формула (6) : Fcn  Expr=-169.72 + 0.605*u(1)
  Формула (8) : Fcn  Expr=1.02+0.0008*u(1)
  Формула №(12) : Fcn  Expr=1/(0.177+0.823*(u(1)/300))^0.4
  Out1 : Outport
  wires:
  Формула №(12)/1 -> Gain2/1
  Формула (8)/1 -> Manual Switch5/1
  Manual Variant Sink/2 -> Формула (10)/1
  Manual Variant Sink1/1 -> Формула (8)/1
  Gain2/1 -> Product/1
  Manual Variant Sink1/2 -> Формула №(12)/1
  Manual Switch5/1 -> Display1/1, Product1/2  "Var"
  " "/1(Out2) -> Scope/1, Out1/1
  Product/1 -> Manual Switch5/2
  Формула (6)/1 -> Manual Switch1/1
  H/1 -> Manual Variant Sink1/1, Manual Variant Sink/1
  V6/1 -> Product/2
  Manual Variant Sink/1 -> Формула (6)/1
  Manual Switch1/1 -> " "/1(Lx), Display2/1
  Формула (10)/1 -> Manual Switch1/2
  Va/1 -> " "/2(Va)
  Product1/1 -> New/1, " "/3("sigma ")
  noise/1 -> Product1/1

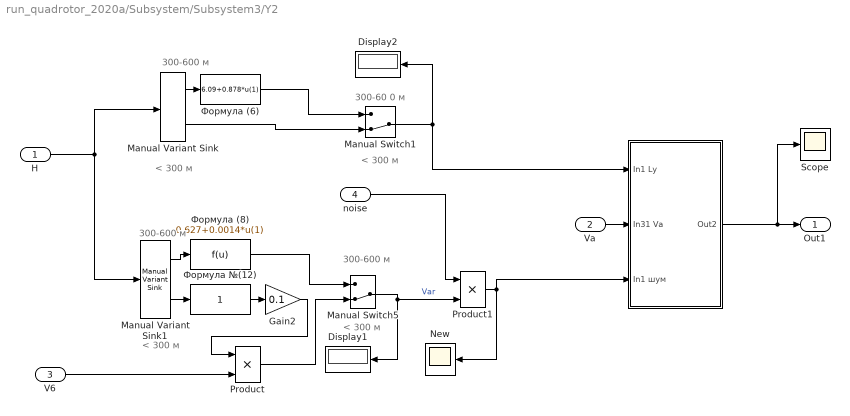
== system run_quadrotor_2020a/Subsystem/Subsystem3/Y2 ==
  note: < 300 м
  note: 300-600 м
  note: < 300 м
  note: < 300 м
  note: 300-600 м
  note: < 300 м
  note: 300-60 0 м
  note: 300-600 м
  H : Inport
  Va : Inport  Port=2
  V6 : Inport  Port=3
  noise : Inport  Port=4
  " " : Subsystem
  Display1 : Display
  Display2 : Display
  Gain2 : Gain  Gain=0.1
  Manual Variant Sink : simulink/Signal Routing/Manual Variant Sink  NumChoices=2  LabelModeActiveChoice=V_2
  Manual Variant Sink1 : simulink/Signal Routing/Manual Variant Sink  NumChoices=2  LabelModeActiveChoice=V_2
  Manual Switch1 : ManualSwitch  CurrentSetting=0
  Manual Switch5 : ManualSwitch  CurrentSetting=0
  New : Scope
  Product : Product
  Product1 : Product
  Scope : Scope
  Формула (6) : Fcn  Expr=6.09+0.878*u(1)
  Формула (8) : Fcn  Expr=0.627+0.0014*u(1)
  Формула №(12) : Fcn  Expr=1
  Out1 : Outport
  wires:
  noise/1 -> Product1/1
  Формула №(12)/1 -> Gain2/1
  Формула (8)/1 -> Manual Switch5/1
  Product1/1 -> New/1, " "/3("In1 шум ")
  Manual Variant Sink1/1 -> Формула (8)/1
  Gain2/1 -> Product/1
  Manual Variant Sink1/2 -> Формула №(12)/1
  Manual Switch5/1 -> Product1/2, Display1/1  "Var"
  " "/1(Out2) -> Scope/1, Out1/1
  Product/1 -> Manual Switch5/2
  Формула (6)/1 -> Manual Switch1/1
  H/1 -> Manual Variant Sink1/1, Manual Variant Sink/1
  V6/1 -> Product/2
  Manual Variant Sink/1 -> Формула (6)/1
  Manual Switch1/1 -> " "/1(In1 Ly), Display2/1
  Manual Variant Sink/2 -> Manual Switch1/2
  Va/1 -> " "/2(In31 Va)

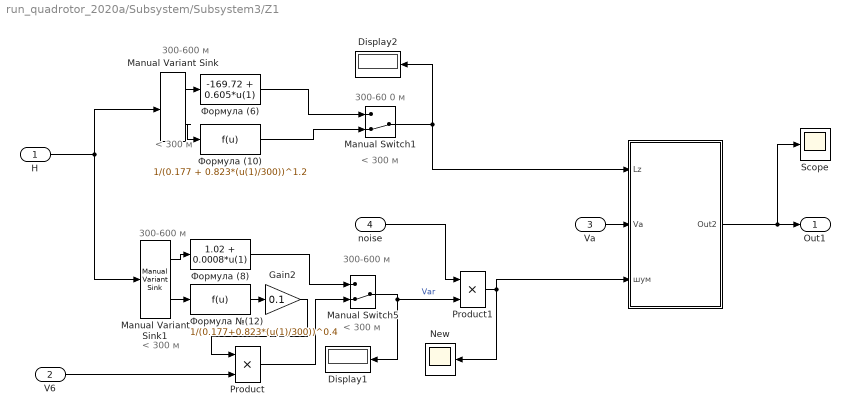
== system run_quadrotor_2020a/Subsystem/Subsystem3/Z1 ==
  note: < 300 м
  note: 300-600 м
  note: < 300 м
  note: < 300 м
  note: 300-600 м
  note: < 300 м
  note: 300-60 0 м
  note: 300-600 м
  H : Inport
  V6 : Inport  Port=2
  Va : Inport  Port=3
  noise : Inport  Port=4
  " " : Subsystem
  Display1 : Display
  Display2 : Display
  Gain2 : Gain  Gain=0.1
  Manual Variant Sink : simulink/Signal Routing/Manual Variant Sink  NumChoices=2  LabelModeActiveChoice=V_2
  Manual Variant Sink1 : simulink/Signal Routing/Manual Variant Sink  NumChoices=2  LabelModeActiveChoice=V_2
  Manual Switch1 : ManualSwitch  CurrentSetting=0
  Manual Switch5 : ManualSwitch  CurrentSetting=0
  New : Scope
  Product : Product
  Product1 : Product
  Scope : Scope
  Формула (10) : Fcn  Expr=1/(0.177 + 0.823*(u(1)/300))^1.2
  Формула (6) : Fcn  Expr=-169.72 + 0.605*u(1)
  Формула (8) : Fcn  Expr=1.02 + 0.0008*u(1)
  Формула №(12) : Fcn  Expr=1/(0.177+0.823*(u(1)/300))^0.4
  Out1 : Outport
  wires:
  noise/1 -> Product1/1
  Формула №(12)/1 -> Gain2/1
  Формула (8)/1 -> Manual Switch5/1
  Product1/1 -> New/1, " "/3("шум ")
  Manual Variant Sink/2 -> Формула (10)/1
  Manual Variant Sink1/1 -> Формула (8)/1
  Gain2/1 -> Product/1
  Manual Variant Sink1/2 -> Формула №(12)/1
  Manual Switch5/1 -> Product1/2, Display1/1  "Var"
  " "/1(Out2) -> Scope/1, Out1/1
  Product/1 -> Manual Switch5/2
  Формула (6)/1 -> Manual Switch1/1
  H/1 -> Manual Variant Sink1/1, Manual Variant Sink/1
  V6/1 -> Product/2
  Manual Variant Sink/1 -> Формула (6)/1
  Manual Switch1/1 -> " "/1(Lz), Display2/1
  Формула (10)/1 -> Manual Switch1/2
  Va/1 -> " "/2(Va)

== system run_quadrotor_2020a/Subsystem/Subsystem3/X1/  ==
  Lx : Inport
  Va : Inport  Port=2
  "sigma " : Inport  Port=3
  Divide3 : Product  Inputs=**
  Divide4 : Product  Inputs=*/
  Fcn3 : Fcn  Expr=u(1)^0.5
  Gain1 : Gain  Gain=2
  Product : Product
  Sum3 : Sum  Inputs=+-
  Transfer Fcn6 : TransferFcn  Denominator="[1  0]"
  Out2 : Outport
  wires:
  Divide4/1 -> [VL], Gain1/1
  Gain1/1 -> Fcn3/1
  Va/1 -> Divide4/1
  Lx/1 -> Divide4/2
  Transfer Fcn6/1 -> Out2/1, Divide3/1  "Драйден фулл"
  Divide3/1 -> Sum3/2
  Sum3/1 -> Transfer Fcn6/1
  [VL] -> Divide3/2
  Product/1 -> Sum3/1  "sigma*Va/Lx)"
  "sigma "/1 -> Product/1
  Fcn3/1 -> Product/2
